simulink model "MPFC_VbyF"  (R2019b)
settings: Solver=ode4  StartTime=0.0  StopTime=1  FixedStep=1e-5  RelTol=1e-3  EnableMultiTasking=on
values from neighbouring files (symbols this model uses):
  B = 0    [Parameters_MPC.m]
  J = 0.0165    [Parameters_MPC.m]
  kr = (Lm/Lr)    (= 0.960714285714)    [Parameters_MPC.m]
  Lm = 0.0538    [Parameters_MPC.m]
  P = 2    [Parameters_MPC.m]
  r_sigma = Rs+Rr*(kr^2)    (= 0.445903864796)    [Parameters_MPC.m]
  Rs = 0.277    [Parameters_MPC.m]
  set_speed = 500    [Parameters_MPC.m]
  t_sigma = (sigma*Ls)/(r_sigma)    (= 0.00810392489023)    [Parameters_MPC.m]
  tr = Lr/Rr    (= 0.306010928962)    [Parameters_MPC.m]
libraries: powerlib_meascontrol x4, simulink x2, powerlib x1
settings Model: Creator=91913  LastModifiedBy=akhil
settings SolverCC: PositivePriorityOrder=on  AutoInsertRateTranBlk=on
settings DataIOCC: SaveOutput=off  DSMLogging=off  ReturnWorkspaceOutputs=off  SignalLoggingName=logsout_MPFC

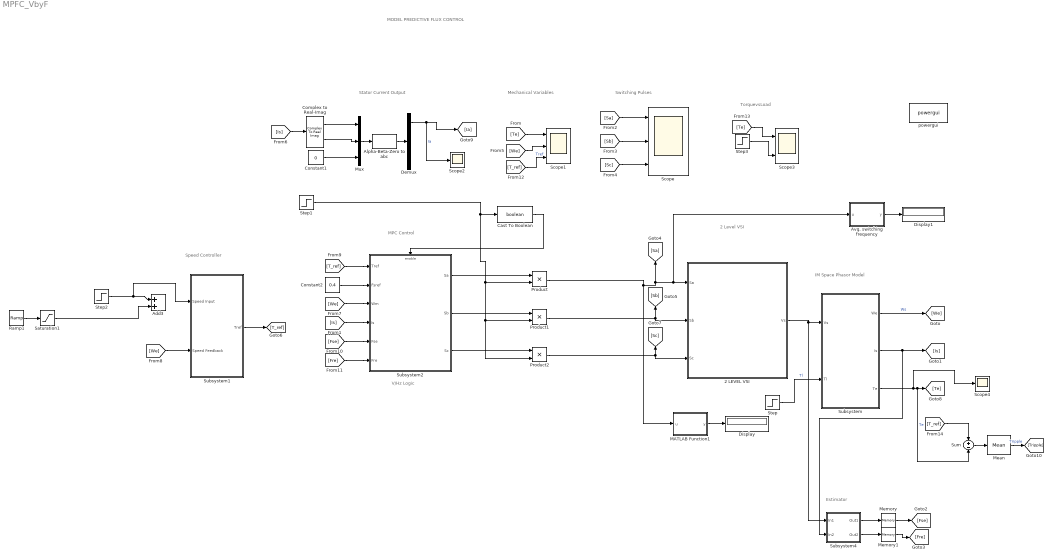
== system MPFC_VbyF ==
  note: MODEL PREDICTIVE FLUX CONTROL
  note: Estimator
  note: V/Hz Logic
  note: Mechanical Variables
  note: Switching Pulses
  note: Speed Controller
  note: 2 Level VSI
  note: MPC Control
  note: IM Space Phasor Model
  note: Stator Current Output
  note: TorquevsLoad
  2 LEVEL VSI : Subsystem
  Add3 : Sum
  Alpha-Beta-Zero to abc : powerlib_meascontrol/Transformations/Alpha-Beta-Zero to abc
      settings: SourceProductName=Simscape Electrical  SourceProductBaseCode=PS
  Avg. switching frequency : MATLAB Function  TreatAsAtomicUnit=on
  Cast To Boolean : DataTypeConversion  OutDataTypeStr=boolean
  Complex to Real-Imag : ComplexToRealImag
  Constant1 : Constant  Value=0
  Constant2 : Constant  Value=0.4
  Demux : Demux  Outputs=3
  Display : Display
  Display1 : Display
  MATLAB Function1 : MATLAB Function  TreatAsAtomicUnit=on
  Mean : powerlib_meascontrol/Measurements/Mean  Freq=40  Vinit=0  Ts=0
      settings: SourceProductName=Simscape Electrical
  Memory : Memory
  Memory1 : Memory
  Mux : Mux  Inputs=3
  Product : Product
  Product1 : Product
  Product2 : Product
  Ramp1 : simulink/Sources/Ramp  slope=-2*set_speed  start=0.4  InitialOutput=0
  Saturation1 : Saturate  UpperLimit=0  LowerLimit=-200
  Scope : Scope  NumInputPorts=3
  Scope1 : Scope  NumInputPorts=3
  Scope2 : Scope
  Scope3 : Scope  NumInputPorts=2
  Scope4 : Scope
  Step : Step  Time=0.5  After=20  SampleTime=0
  Step1 : Step  Time=0  SampleTime=0
  Step2 : Step  Time=0.1  After=set_speed  SampleTime=0
  Step3 : Step  Time=3.5  After=20  SampleTime=0
  Subsystem : Subsystem
  Subsystem1 : Subsystem
  Subsystem2 : Subsystem
  Subsystem4 : Subsystem
  Sum : Sum  Inputs=+-
  powergui : powerlib/powergui  Priority=1  SimulationMode=Continuous  SampleTime=50e-6  frequency=60  Iterations=50  frequencyindice=60  Pbase=100e6  ErrMax=1e-4  UnitsV=kV  UnitsW=MW  buscounter=0  FunctionMessages=off  echomessages=off  EnableUseOfTLC=off  CurrentSourceSwitches=off  DisableSnubberDevices=off  DisableRonSwitches=off  DisableVfSwitches=off  DisplayEquations=off  AutomaticDiscreteSolvers=off  SolverType=Tustin/Backward Euler (TBE)  Interpol=off  ExternalGateDelay=off  methode=off  Ts=100  x0status=blocks  SPID=on  SwTol=0  HookPort=off  NonlinearTolerance=1e-4  nMaxIteration=100  ContinueOnMaxIteration=off  RestoreLinks=warning  ResistiveCurrentMeasurement=off  Frange=[0:2:500]  Ylog=off  Xlog=on  ShowGrid=off  save=off  variable=ZData  structure=logsout_MPFC  ZoomFFT=off  StartTime=0.6  cycles=10  DisplayStyle=1  fundamental=49.26  FreqAxis=on  MaxFrequency=2000  frequencyindicesteady=1  RmsSteady=1  display=off
      settings: SourceProductName=Simscape Electrical
  wires:
  Subsystem/1(We) -> [We]  "Ws"
  Subsystem/2(Is) -> [Is], Subsystem4/2(In2)
  [Sa] -> Scope/1
  [Sb] -> Scope/2
  [Sc] -> Scope/3
  [Te] -> Scope1/1
  [We] -> Scope1/2
  [Is] -> Complex to Real-Imag/1
  Complex to Real-Imag/2 -> Mux/2
  Constant1/1 -> Mux/3
  Mux/1 -> Alpha-Beta-Zero to abc/1
  Complex to Real-Imag/1 -> Mux/1
  Alpha-Beta-Zero to abc/1 -> Demux/1
  Demux/1 -> Scope2/1, [Ia]  "Ia"
  [We] -> Subsystem1/2(Speed Feedback)
  [T_ref] -> Scope1/3  "Tref"
  Constant2/1 -> Subsystem2/2(Fsref)
  [We] -> Subsystem2/3(Wm)
  [Is] -> Subsystem2/4(Is)
  Subsystem2/1(Sa) -> Product/1
  Subsystem2/2(Sb) -> Product1/1
  Subsystem2/3(Sc) -> Product2/1
  2 LEVEL VSI/1(Vs) -> Subsystem/1(Vs), Subsystem4/1(In1)
  Step1/1 -> Product2/2, Product1/2, Product/2, Cast To Boolean/1
  Product/1 -> MATLAB Function1/1(u), [Sa], Avg. switching frequency/1(u), 2 LEVEL VSI/1(Sa)
  Product1/1 -> 2 LEVEL VSI/2(Sb), [Sb]
  Product2/1 -> 2 LEVEL VSI/3(Sc), [Sc]
  Cast To Boolean/1 -> Subsystem2/Enable
  Subsystem1/1(Tref) -> [T_ref]
  Step3/1 -> Scope3/2
  [Te] -> Scope3/1
  Subsystem4/1(Out1) -> Memory/1
  Subsystem4/2(Out2) -> Memory1/1
  Memory/1 -> [Fse]
  Memory1/1 -> [Fre]
  [Fse] -> Subsystem2/5(Fse)
  [Fre] -> Subsystem2/6(Fre)
  Subsystem/3(Te) -> Scope4/1, Sum/2, [Te]  "Te"
  [T_ref] -> Sum/1
  Sum/1 -> Mean/1
  Mean/1 -> [Tripple]  "Tripple"
  [T_ref] -> Subsystem2/1(Tref)
  Step/1 -> Subsystem/2(Tl)  "Tl"
  MATLAB Function1/1(y) -> Display/1
  Avg. switching frequency/1(y) -> Display1/1
  Saturation1/1 -> Add3/2
  Step2/1 -> Subsystem1/1(Speed Input), Add3/1
  Ramp1/1 -> Saturation1/1

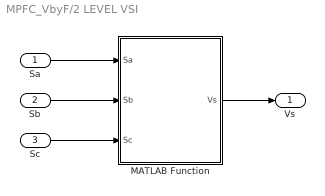
== system MPFC_VbyF/2 LEVEL VSI ==
  Sa : Inport
  Sb : Inport  Port=2
  Sc : Inport  Port=3
  MATLAB Function : MATLAB Function  TreatAsAtomicUnit=on
  Vs : Outport
  wires:
  Sa/1 -> MATLAB Function/1(Sa)
  MATLAB Function/1(Vs) -> Vs/1
  Sb/1 -> MATLAB Function/2(Sb)
  Sc/1 -> MATLAB Function/3(Sc)

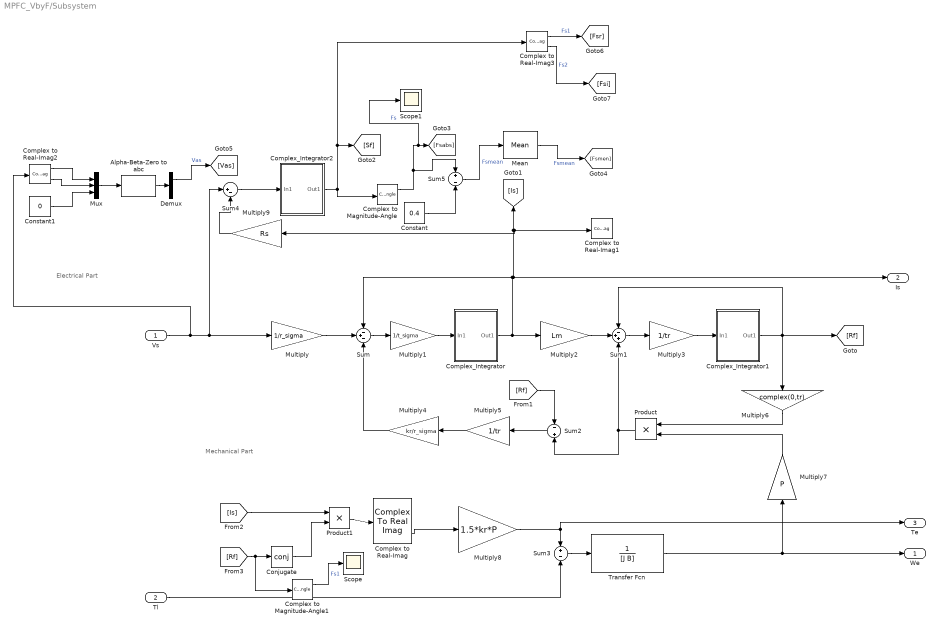
== system MPFC_VbyF/Subsystem ==
  note: Mechanical Part
  note: Electrical Part
  Vs : Inport
  Tl : Inport  Port=2
  Alpha-Beta-Zero to abc : powerlib_meascontrol/Transformations/Alpha-Beta-Zero to abc
      settings: SourceProductName=Simscape Electrical  SourceProductBaseCode=PS
  Complex to Magnitude-Angle : ComplexToMagnitudeAngle
  Complex to Magnitude-Angle1 : ComplexToMagnitudeAngle
  Complex to Real-Imag{,1..3} (4 alike) : ComplexToRealImag
  Complex_Integrator : Subsystem
  Complex_Integrator1 : Subsystem
  Complex_Integrator2 : Subsystem
  Conjugate : Math  Operator=conj  RndMeth=Zero  SaturateOnIntegerOverflow=on
  Constant : Constant  Value=0.4
  Constant1 : Constant  Value=0
  Demux : Demux  Outputs=3
  Mean : powerlib_meascontrol/Measurements/Mean  Freq=40  Vinit=0  Ts=0
      settings: SourceProductName=Simscape Electrical
  Multiply : Gain  Gain=1/r_sigma
  Multiply1 : Gain  Gain=1/t_sigma
  Multiply2 : Gain  Gain=Lm
  Multiply3 : Gain  Gain=1/tr
  Multiply4 : Gain  Gain=kr/r_sigma
  Multiply5 : Gain  Gain=1/tr
  Multiply6 : Gain  Gain=complex(0,tr)
  Multiply7 : Gain  Gain=P
  Multiply8 : Gain  Gain=1.5*kr*P
  Multiply9 : Gain  Gain=Rs
  Mux : Mux  Inputs=3
  Product : Product
  Product1 : Product
  Scope : Scope
  Scope1 : Scope
  Sum : Sum  Inputs=-+-
  Sum1 : Sum  Inputs=-++
  Sum2 : Sum  Inputs=-+
  Sum3 : Sum  Inputs=+-
  Sum4 : Sum  Inputs=|+-
  Sum5 : Sum  Inputs=+-
  Transfer Fcn : TransferFcn  Denominator=[J B]
  We : Outport
  Is : Outport  Port=2
  Te : Outport  Port=3
  wires:
  [Is] -> Product1/1
  Multiply1/1 -> Complex_Integrator/1(In1)
  Multiply4/1 -> Sum/3
  Multiply3/1 -> Complex_Integrator1/1(In1)
  Sum1/1 -> Multiply3/1
  Complex to Real-Imag/2 -> Multiply8/1
  Complex_Integrator1/1(Out1) -> Sum1/1, [Rf], Multiply6/1
  Tl/1 -> Sum3/2
  Conjugate/1 -> Product1/2
  Multiply7/1 -> Product/2
  Multiply8/1 -> Sum3/1, Te/1
  Multiply2/1 -> Sum1/2
  Multiply/1 -> Sum/2
  Multiply6/1 -> Product/1
  Product/1 -> Sum2/2, Sum1/3
  Complex_Integrator/1(Out1) -> Multiply2/1, Multiply9/1, Complex to Real-Imag1/1, [Is], Is/1, Sum/1
  Multiply5/1 -> Multiply4/1
  Sum2/1 -> Multiply5/1
  Vs/1 -> Complex to Real-Imag2/1, Sum4/1, Multiply/1
  Transfer Fcn/1 -> We/1, Multiply7/1
  Sum/1 -> Multiply1/1
  [Rf] -> Complex to Magnitude-Angle1/1, Conjugate/1
  Product1/1 -> Complex to Real-Imag/1
  Sum3/1 -> Transfer Fcn/1
  [Rf] -> Sum2/1
  Multiply9/1 -> Sum4/2
  Sum4/1 -> Complex_Integrator2/1(In1)
  Complex_Integrator2/1(Out1) -> Complex to Magnitude-Angle/1, Complex to Real-Imag3/1, [Sf]
  Complex to Magnitude-Angle/1 -> Sum5/1, Scope1/1, [Fsabs]  "Fs"
  Constant/1 -> Sum5/2
  Sum5/1 -> Mean/1  "Fsmean"
  Mean/1 -> [Fsmen]  "Fsmean"
  Complex to Real-Imag2/1 -> Mux/1
  Complex to Real-Imag2/2 -> Mux/2
  Constant1/1 -> Mux/3
  Mux/1 -> Alpha-Beta-Zero to abc/1
  Alpha-Beta-Zero to abc/1 -> Demux/1
  Demux/1 -> [Vas]  "Vas"
  Complex to Magnitude-Angle1/1 -> Scope/1  "Fs1"
  Complex to Real-Imag3/2 -> [Fsi]  "Fs2"
  Complex to Real-Imag3/1 -> [Fsr]  "Fs1"

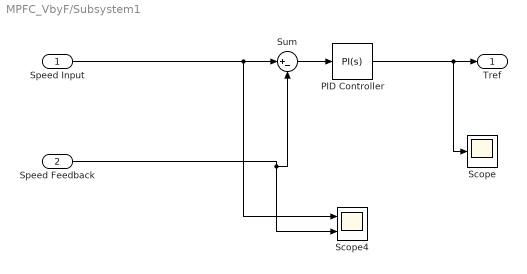
== system MPFC_VbyF/Subsystem1 ==
  Speed Input : Inport
  Speed Feedback : Inport  Port=2
  PID Controller : simulink/Continuous/PID Controller  Controller=PI  Form=Parallel  TimeDomain=Continuous-time  SampleTime=-1  IntegratorMethod=Forward Euler  FilterMethod=Forward Euler  ControllerParametersSource=internal  P=100  I=2000  D=0  UseFilter=on  N=100  TunerSelectOption=Transfer Function Based (PID Tuner App)  InitialConditionSource=internal  InitialConditionForIntegrator=0  InitialConditionForFilter=0  DifferentiatorICPrevScaledInput=0  ExternalReset=none  TrackingMode=off  Kt=1  LimitOutput=on  UpperSaturationLimit=30  LowerSaturationLimit=-30  LinearizeAsGain=on  AntiWindupMode=clamping  Kb=1  POutMin=[]  POutMax=[]  IOutMin=[]  IOutMax=[]  DOutMin=[]  DOutMax=[]  NOutMin=[]  NOutMax=[]  SumOutMin=[]  SumOutMax=[]  SaturationOutMin=[]  SaturationOutMax=[]  PParamMin=[]  PParamMax=[]  IParamMin=[]  IParamMax=[]  DParamMin=[]  DParamMax=[]  NParamMin=[]  NParamMax=[]  KbParamMin=[]  KbParamMax=[]  KtParamMin=[]  KtParamMax=[]  KbOutMin=[]  KbOutMax=[]  KtOutMin=[]  KtOutMax=[]  IntegratorOutMin=[]  IntegratorOutMax=[]  FilterOutMin=[]  FilterOutMax=[]  SumI1OutMin=[]  SumI1OutMax=[]  SumI2OutMin=[]  SumI2OutMax=[]  SumI3OutMin=[]  SumI3OutMax=[]  SumI4OutMin=[]  SumI4OutMax=[]  SumDOutMin=[]  SumDOutMax=[]  DifferentiatorOutMin=[]  DifferentiatorOutMax=[]  FilterDiffOutCoefMin=[]  FilterDiffOutCoefMax=[]  ReciprocalOutMin=[]  ReciprocalOutMax=[]  SumDenOutMin=[]  SumDenOutMax=[]  SumNumOutMin=[]  SumNumOutMax=[]  DivideOutMin=[]  DivideOutMax=[]  IntegratorContinuousStateAttributes=''  IntegratorStateMustResolveToSignalObject=off  IntegratorRTWStateStorageClass=Auto  FilterContinuousStateAttributes=''  FilterStateMustResolveToSignalObject=off  FilterRTWStateStorageClass=Auto  ParallelPVariant=InternalParameters  IdealPVariant=Disabled  IVariant=InternalParameters  DVariant=Disabled  IntegratorVariant=Continuous  SatVariant=Enabled  AWVariant=ContClampingParallel  PCopyVariant=Disabled  TRVariant=Disabled  FdbkBlocksVariant=Forward  IdealPFdbkVariant=Disabled  SatFdbkVariant=Disabled  DerivativeFilterVariant=Disabled  NVariant=Disabled  NCopyVariant=Disabled_SignalSpec  FilterICVariant=Disabled  IntegratorICVariant=InternalICs  ExternalResetVariant=Disabled  TRSumVariant=Passthrough  SumFdbkVariant=Disabled  SumVariant=Sum_PI
  Scope : Scope
  Scope4 : Scope  NumInputPorts=2
  Sum : Sum  Inputs=|+-
  Tref : Outport
  wires:
  Speed Input/1 -> Scope4/1, Sum/1
  Speed Feedback/1 -> Scope4/2, Sum/2
  Sum/1 -> PID Controller/1
  PID Controller/1 -> Scope/1, Tref/1

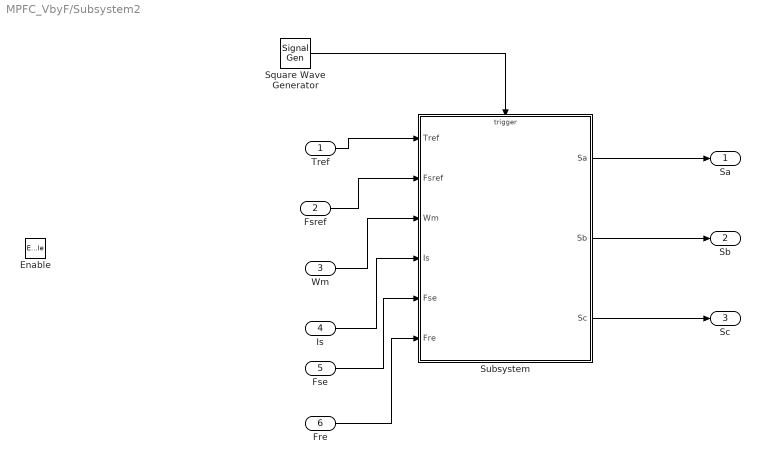
== system MPFC_VbyF/Subsystem2 ==
  Tref : Inport
  Fsref : Inport  Port=2
  Wm : Inport  Port=3
  Is : Inport  Port=4
  Fse : Inport  Port=5
  Fre : Inport  Port=6
  Enable : EnablePort
  Square Wave Generator : SignalGenerator  WaveForm=square  Frequency=1/50e-6
  Subsystem : Subsystem
  Sa : Outport
  Sb : Outport  Port=2
  Sc : Outport  Port=3
  wires:
  Tref/1 -> Subsystem/1(Tref)
  Fsref/1 -> Subsystem/2(Fsref)
  Wm/1 -> Subsystem/3(Wm)
  Is/1 -> Subsystem/4(Is)
  Fse/1 -> Subsystem/5(Fse)
  Fre/1 -> Subsystem/6(Fre)
  Subsystem/1(Sa) -> Sa/1
  Subsystem/2(Sb) -> Sb/1
  Subsystem/3(Sc) -> Sc/1
  Square Wave Generator/1 -> Subsystem/Trigger

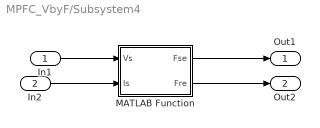
== system MPFC_VbyF/Subsystem4 ==
  In1 : Inport
  In2 : Inport  Port=2
  MATLAB Function : MATLAB Function  TreatAsAtomicUnit=on
  Out1 : Outport
  Out2 : Outport  Port=2
  wires:
  In1/1 -> MATLAB Function/1(Vs)
  In2/1 -> MATLAB Function/2(Is)
  MATLAB Function/2(Fre) -> Out2/1
  MATLAB Function/1(Fse) -> Out1/1

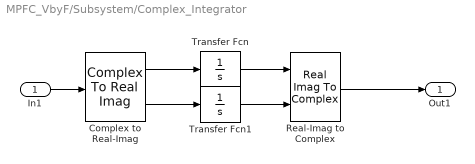
== system MPFC_VbyF/Subsystem/Complex_Integrator ==
  In1 : Inport
  Complex to Real-Imag : ComplexToRealImag
  Real-Imag to Complex : RealImagToComplex
  Transfer Fcn : TransferFcn  Denominator=[1 0]
  Transfer Fcn1 : TransferFcn  Denominator=[1 0]
  Out1 : Outport
  wires:
  In1/1 -> Complex to Real-Imag/1
  Complex to Real-Imag/1 -> Transfer Fcn/1
  Complex to Real-Imag/2 -> Transfer Fcn1/1
  Transfer Fcn/1 -> Real-Imag to Complex/1
  Transfer Fcn1/1 -> Real-Imag to Complex/2
  Real-Imag to Complex/1 -> Out1/1

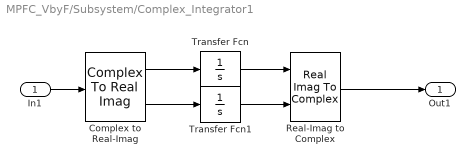
== system MPFC_VbyF/Subsystem/Complex_Integrator1 ==
  In1 : Inport
  Complex to Real-Imag : ComplexToRealImag
  Real-Imag to Complex : RealImagToComplex
  Transfer Fcn : TransferFcn  Denominator=[1 0]
  Transfer Fcn1 : TransferFcn  Denominator=[1 0]
  Out1 : Outport
  wires:
  In1/1 -> Complex to Real-Imag/1
  Complex to Real-Imag/1 -> Transfer Fcn/1
  Complex to Real-Imag/2 -> Transfer Fcn1/1
  Transfer Fcn/1 -> Real-Imag to Complex/1
  Transfer Fcn1/1 -> Real-Imag to Complex/2
  Real-Imag to Complex/1 -> Out1/1

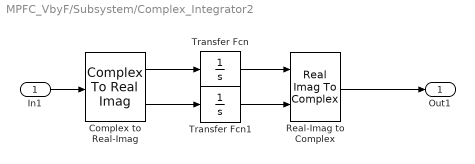
== system MPFC_VbyF/Subsystem/Complex_Integrator2 ==
  In1 : Inport
  Complex to Real-Imag : ComplexToRealImag
  Real-Imag to Complex : RealImagToComplex
  Transfer Fcn : TransferFcn  Denominator=[1 0]
  Transfer Fcn1 : TransferFcn  Denominator=[1 0]
  Out1 : Outport
  wires:
  In1/1 -> Complex to Real-Imag/1
  Complex to Real-Imag/1 -> Transfer Fcn/1
  Complex to Real-Imag/2 -> Transfer Fcn1/1
  Transfer Fcn/1 -> Real-Imag to Complex/1
  Transfer Fcn1/1 -> Real-Imag to Complex/2
  Real-Imag to Complex/1 -> Out1/1

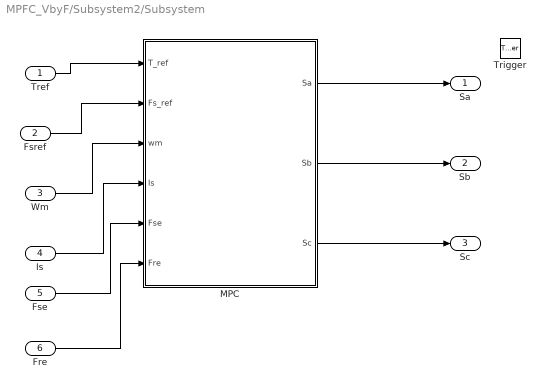
== system MPFC_VbyF/Subsystem2/Subsystem ==
  Tref : Inport
  Fsref : Inport  Port=2
  Wm : Inport  Port=3
  Is : Inport  Port=4
  Fse : Inport  Port=5
  Fre : Inport  Port=6
  Trigger : TriggerPort  VariantControl=Variant  PortDimensions=1
  MPC : MATLAB Function  TreatAsAtomicUnit=on
  Sa : Outport
  Sb : Outport  Port=2
  Sc : Outport  Port=3
  wires:
  Fsref/1 -> MPC/2(Fs_ref)
  Tref/1 -> MPC/1(T_ref)
  Fre/1 -> MPC/6(Fre)
  Wm/1 -> MPC/3(wm)
  Is/1 -> MPC/4(Is)
  Fse/1 -> MPC/5(Fse)
  MPC/1(Sa) -> Sa/1
  MPC/2(Sb) -> Sb/1
  MPC/3(Sc) -> Sc/1

== matlab function MPFC_VbyF/Subsystem2/Subsystem/MPC ==
  settings: updateMethod=DISCRETE
  data: T_ref input; Sa output; Fs_ref input; wm input; Is input; Sb output; Sc output; Fse input; Fre input
function [Sa,Sb,Sc]   = MPC(T_ref,Fs_ref,wm,Is,Fse,Fre)

Ts=50e-6;%Sampling time or Time Window for Kth sample
%Supply DC Voltage
Vdc=250;
%Machine Parameters
Rs=0.277;
Rr=0.183;
Lr=0.056;
Ls=0.0553;
Lm=0.0538;
P=2;%pole pairs
Is_nom=25;
%Electrical Time Constants
tr=Lr/Rr;
%Constants in equation
sigma=(1-(Lm^2)/(Ls*Lr));
kr=(Lm/Lr);
r_sigma=Rs+Rr*(kr^2);
t_sigma=(sigma*Ls)/(r_sigma);
delta=1/((Ls*Lr)-Lm^2);
%weight=T_nom/Fs_nom;
%Voltage vectors
V0=0;
V1=complex((2/3)*Vdc,0);
V2=complex((1/3)*Vdc,(sqrt(3)/3)*Vdc);
V3=complex((-1/3)*Vdc,(sqrt(3)/3)*Vdc);
V4=-V1;
V5=-V2;
V6=-V3;
V7= V0;
V=[V0 V1 V2 V3 V4 V5 V6 V7];
%Switching States

states=[0 0 0;1 0 0;1 1 0;0 1 0;0 1 1;0 0 1;1 0 1;1 1 1];

persistent x_opt  %since previous values are required for prediction and estimation
if isempty(x_opt)
    x_opt=2;
end


[theta, rho] = cart2pol(real(Fre), imag(Fre));
cost_opt=1e14;
   
if(abs(T_ref)/(1.5*delta*Lm*rho*Fs_ref*P)>1 )
angle_ref=pi/2;    
else
angle_ref=theta+asin((T_ref)/(1.5*delta*Lm*rho*Fs_ref*P));
end
Fs_ref1=0;
if(Fs_ref~=0.4)
Fs_ref1=0.4;
else
Fs_ref1=0.4;
end
Fsref=Fs_ref1*exp(1i*angle_ref);
%Prediction of stator current,flux vectors and Torque for each voltage
%vectors
for loop=1:8
    
    V_loop=V(loop);% iterative voltage vector
      %Stator current prediction
    Isp=Is*(t_sigma/(Ts+t_sigma))+(Ts/(t_sigma+Ts))*(1/r_sigma)*(Fre*((kr/tr)-complex(0,wm*kr))+V_loop);
    %Stator flux prediction based on discretization
    Fsp=Fse+(Ts*V_loop)-Rs*Ts*Isp;
  
      f=0;
      if abs(Isp) > Is_nom  
            f = 1e14; 
            
      end
      cost=abs(Fsref-Fsp)+f;
     if(cost<cost_opt) 
     x_opt=loop;
     cost_opt=cost;
     end     
end
%Outpt switching states
Sa=states(x_opt,1);
Sb=states(x_opt,2);
Sc=states(x_opt,3);

== matlab function MPFC_VbyF/2 LEVEL VSI/MATLAB Function ==
  data: Sa input; Vs output; Sb input; Sc input
function Vs = fcn(Sa,Sb,Sc)
Vdc=250;
a=complex(cos(2*pi/3),sin(2*pi/3)); 
Vs =(2/3)*Vdc*(Sa+(a*Sb)+((a^2)*Sc)) ;

== matlab function MPFC_VbyF/Subsystem4/MATLAB Function ==
  settings: updateMethod=DISCRETE
  data: Vs input; Fse output; Is input; Fre output
function [Fse,Fre] = fcn(Vs,Is)

Ts=1e-5;%Sampling time or Time Window for Kth sample
%Supply DC Voltage
%Machine Parameters
Rs=0.277;
Lr=0.056;
Ls=0.0553;
Lm=0.0538;

persistent  Fs

if isempty(Fs)
    Fs=complex(0,0);
end

%stator flux estimate
Fs=Fs+Ts*(Vs-(Rs*Is)); 
%Rotor Flux estimate
Fre=(Lr/Lm)*Fs+Is*(Lm-(Lr*Ls/Lm));
Fse=Fs;

== matlab function MPFC_VbyF/MATLAB Function1 ==
  settings: updateMethod=DISCRETE
  data: u input; y output
function y = fcn(u)
persistent count prestate;
if(isempty(count))
    count=0;
end    
if(isempty(prestate))
    prestate=0;
end  
if(u~=prestate)
count=count+1;    
end
prestate=u;
y=count;

== matlab function MPFC_VbyF/Avg. switching frequency ==
  settings: updateMethod=DISCRETE
  data: u input; y output
function y = fcn(u)
persistent count prestate;
if(isempty(count))
    count=0;
end    
if(isempty(prestate))
    prestate=0;
end  
if(u~=prestate)
count=count+1;    
end
prestate=u;
y=count;
